simulink model "puzzlebot_controladores"  (R2024a)
settings: Solver=VariableStepAuto  StartTime=0.0  StopTime=220  RelTol=1e-3
libraries: slpidlib x2
settings Model: Creator=KALED  LastModifiedBy=KALED

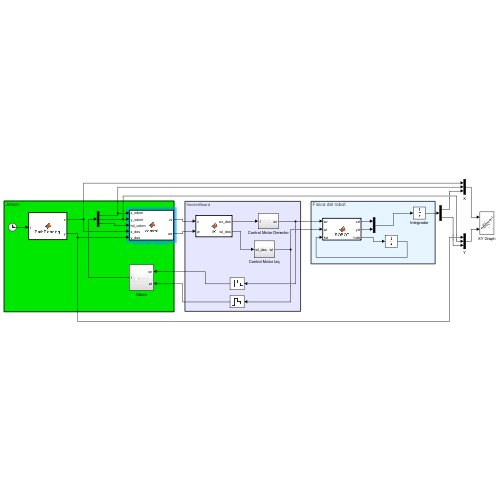
[thumbnail: Simulink's stored preview of the top-level diagram]
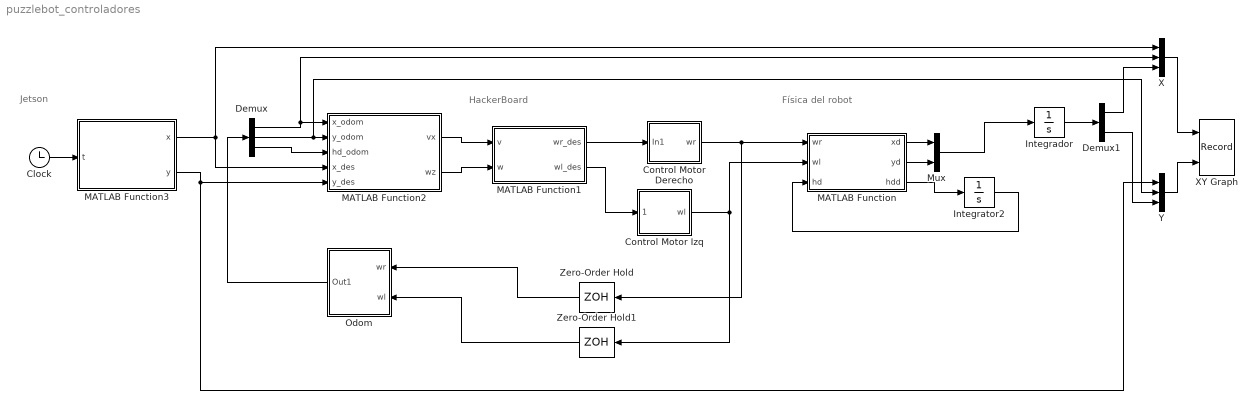
== system puzzlebot_controladores ==
  note: Jetson
  note: HackerBoard
  note: Física del robot
  Clock : Clock
  Control Motor Derecho : Subsystem
  Control Motor Izq : Subsystem
  Demux : Demux  Outputs=3
  Demux1 : Demux  Outputs=2
  Integrador : Integrator  InitialCondition=[0,0]
  Integrator2 : Integrator  ContinuousStateAttributes='orientation'
  MATLAB Function : MATLAB Function  TreatAsAtomicUnit=on
  MATLAB Function1 : MATLAB Function  TreatAsAtomicUnit=on
  MATLAB Function2 : MATLAB Function  TreatAsAtomicUnit=on
  MATLAB Function3 : MATLAB Function  TreatAsAtomicUnit=on
  Mux : Mux  Inputs=2
  Odom : Subsystem
  X : Mux  Inputs=3
  XY Graph : Record  FileSettingsInternal="{\"entries\":[{\"content\":{\"excelSettings\":{\"content\":{},\"type\":\"Streamout.ExcelSettings\"}},\"type\":\"Streamout.FileSettingStorage\",\"uuid\":\"\"}],\"packageUris\":[\"http:\\/\\/schema.mathworks.com\\/mf0\\/streamout_blocks\\/R2020a\"],\"version\":\"1.0\"}"  Layout=[1 1]  SignalsInternal="{\"entries\":[{\"content\":{\"signals\":[{\"content\":{\"blockPath\":[],\"dimensions\":[3],\"domain\":\"\",\"hasChildren\":true,\"lineColor\":\"#fe330a\",\"lineWidth\":2,\"port\":1,\"sid\":[\"\"],\"signalID\":1,\"signalName\":\"X\"},\"type\":\"RecordBlkView.Signal\",\"uuid\":\"\"},{\"content\":{\"blockPath\":[],\"channel\":[1],\"dimensions\":[3],\"domain\":\"\",\"lineColor\":\"#139fff\",\"parentID\":1,\"plots\":[ 1 ],\"port\":1,\"sid\":[\"\"],\"signalID\":2,\"signalName\":\"X\"},\"type\":\"RecordBlkView.Signal\",\"uuid\":\"\"},{\"content\":{\"blockPath\":[],\"dimensions\":[3],\"domain\":\"\",\"hasChildren\":true,\"lineColor\":\"#0072bd\",\"lineWidth\":2,\"port\":2,\"sid\":[\"\"],\"signalID\":3,\"signalName\":\"Y\"},\"type\":\"RecordBlkView.Signal\",\"uuid\":\"\"},{\"content\":{\"blockPath\":[],\"channel\":[1],\"dimensions\":[3],\"domain\":\"\",\"lineColor\":\"#b746ff\",\"parentID\":3,\"plots\":[ 1 ],\"port\":2,\"sid\":[\"\"],\"signalID\":4,\"signalName\":\"Y\"},\"type\":\"RecordBlkView.Signal\",\"uuid\":\"\"},{\"content\":{\"blockPath\":[],\"channel\":[2],\"dimensions\":[3],\"domain\":\"\",\"lineColor\":\"#64d413\",\"parentID\":1,\"plots\":[ 1 ],\"port\":1,\"sid\":[\"\"],\"signalID\":5,\"signalName\":\"X\"},\"type\":\"RecordBlkView.Signal\",\"uuid\":\"\"},{\"content\":{\"blockPath\":[],\"channel\":[3],\"dimensions\":[3],\"domain\":\"\",\"lineColor\":\"#ff6929\",\"lineWidth\":2,\"parentID\":1,\"plots\":[ 1 ],\"port\":1,\"sid\":[\"\"],\"signalID\":6,\"signalName\":\"X\"},\"type\":\"RecordBlkView.Signal\",\"uuid\":\"\"},{\"content\":{\"blockPath\":[],\"channel\":[2],\"dimensions\":[3],\"domain\":\"\",\"lineColor\":\"#ff13a6\",\"parentID\":3,\"plots\":[ 1 ],\"port\":2,\"sid\":[\"\"],\"signalID\":7,\"signalName\":\"Y\"},\"type\":\"RecordBlkView.Signal\",\"uuid\":\"\"},{\"content\":{\"blockPath\":[],\"channel\":[3],\"dimensions\":[3],\"domain\":\"\",\"lineColor\":\"#64d413\",\"lineWidth\":2,\"parentID\":3,\"plots\":[ 1 ],\"port\":2,\"sid\":[\"\"],\"signalID\":8,\"signalName\":\"Y\"},\"type\":\"RecordBlkView.Signal\",\"uuid\":\"\"}]},\"type\":\"RecordBlkView.InputSignals\",\"uuid\":\"\"}],\"packageUris\":[\"http:\\/\\/schema.mathworks.com\\/mf0\\/streamout_blocks\\/R2020a\"],\"version\":\"1.0\"}"  VisualizationBindings="{\"xyplotplugin\":{\"info\":[{\"series\":[{\"bindingParametersList\":[{\"parameter\":\"X-Axis\",\"signalID\":6,\"signalName\":\"X(3)\"},{\"parameter\":\"Y-Axis\",\"signalID\":8,\"signalName\":\"Y(3)\"}],\"seriesID\":0},{\"bindingParametersList\":[{\"parameter\":\"X-Axis\",\"signalID\":2,\"signalName\":\"X(1)\"},{\"parameter\":\"Y-Axis\",\"signalID\":4,\"signalName\":\"Y(1)\"}],\"seriesID\":1},{\"bindingParametersList\":[{\"parameter\":\"X-Axis\",\"signalID\":5,\"signalName\":\"X(2)\"},{\"parameter\":\"Y-Axis\",\"signalID\":7,\"signalName\":\"Y(2)\"}],\"seriesID\":2}],\"subplotID\":1}]}}"  CompatibilityTag=XY
  Y : Mux  Inputs=3
  Zero-Order Hold : ZeroOrderHold  SampleTime=0.01
  Zero-Order Hold1 : ZeroOrderHold  SampleTime=0.01
  wires:
  Odom/1(Out1) -> Demux/1
  X/1 -> XY Graph/1
  Demux1/2 -> Y/3
  Demux/2 -> Y/2, MATLAB Function2/2(y_odom)
  Zero-Order Hold/1 -> Odom/1(wr)
  Demux1/1 -> X/3
  MATLAB Function1/2(wl_des) -> Control Motor Izq/1(wl_des)
  MATLAB Function/3(hdd) -> Integrator2/1
  Integrator2/1 -> MATLAB Function/3(hd)
  Control Motor Derecho/1(wr) -> Zero-Order Hold/1, MATLAB Function/1(wr)
  MATLAB Function1/1(wr_des) -> Control Motor Derecho/1(In1)
  MATLAB Function/1(xd) -> Mux/1
  Integrador/1 -> Demux1/1
  MATLAB Function3/1(x) -> X/1, MATLAB Function2/4(x_des)
  MATLAB Function2/2(wz) -> MATLAB Function1/2(w)
  Mux/1 -> Integrador/1
  MATLAB Function3/2(y) -> Y/1, MATLAB Function2/5(y_des)
  Zero-Order Hold1/1 -> Odom/2(wl)
  MATLAB Function2/1(vx) -> MATLAB Function1/1(v)
  Clock/1 -> MATLAB Function3/1(t)
  Demux/3 -> MATLAB Function2/3(hd_odom)
  MATLAB Function/2(yd) -> Mux/2
  Demux/1 -> X/2, MATLAB Function2/1(x_odom)
  Control Motor Izq/1(wl) -> MATLAB Function/2(wl), Zero-Order Hold1/1
  Y/1 -> XY Graph/2

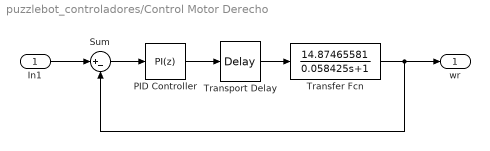
== system puzzlebot_controladores/Control Motor Derecho ==
  In1 : Inport
  PID Controller : slpidlib/PID Controller  Controller=PI  Form=Parallel  TimeDomain=Discrete-time  UseExternalTs=off  SampleTime=0.01  IntegratorMethod=Forward Euler  FilterMethod=Forward Euler  ControllerParametersSource=internal  P=0.03143  I=0.22281  UseKiTs=off  D=0  UseExternalDerivativeSource=off  N=100  UseFilter=on  TunerSelectOption=Transfer Function Based (PID Tuner App)  InitialConditionSource=internal  InitialConditionForIntegrator=0  InitialConditionForFilter=0  DifferentiatorICPrevScaledInput=0  ExternalReset=none  TrackingMode=off  Kt=1  LimitOutput=on  SatLimitsSource=internal  UpperSaturationLimit=1  LowerSaturationLimit=-1  LinearizeAsGain=on  AntiWindupMode=none  Kb=1  LimitIntegrator=off  UpperIntegratorSaturationLimit=inf  LowerIntegratorSaturationLimit=-inf  POutMin=[]  POutMax=[]  IOutMin=[]  IOutMax=[]  DOutMin=[]  DOutMax=[]  NOutMin=[]  NOutMax=[]  SumOutMin=[]  SumOutMax=[]  SaturationOutMin=[]  SaturationOutMax=[]  PParamMin=[]  PParamMax=[]  IParamMin=[]  IParamMax=[]  DParamMin=[]  DParamMax=[]  NParamMin=[]  NParamMax=[]  KbParamMin=[]  KbParamMax=[]  KtParamMin=[]  KtParamMax=[]  KbOutMin=[]  KbOutMax=[]  KtOutMin=[]  KtOutMax=[]  IntegratorOutMin=[]  IntegratorOutMax=[]  FilterOutMin=[]  FilterOutMax=[]  SumI1OutMin=[]  SumI1OutMax=[]  SumI2OutMin=[]  SumI2OutMax=[]  SumI3OutMin=[]  SumI3OutMax=[]  SumI4OutMin=[]  SumI4OutMax=[]  SumDOutMin=[]  SumDOutMax=[]  DifferentiatorOutMin=[]  DifferentiatorOutMax=[]  FilterDiffOutCoefMin=[]  FilterDiffOutCoefMax=[]  ReciprocalOutMin=[]  ReciprocalOutMax=[]  SumDenOutMin=[]  SumDenOutMax=[]  SumNumOutMin=[]  SumNumOutMax=[]  DivideOutMin=[]  DivideOutMax=[]  UdiffTsProdOutMin=[]  UdiffTsProdOutMax=[]  NTsProdOutMin=[]  NTsProdOutMax=[]  UintegralTsProdOutMin=[]  UintegralTsProdOutMax=[]  UngainTsProdOutMin=[]  UngainTsProdOutMax=[]  ClampingZeroOutDataTypeStr=Inherit: Inherit via back propagation  ClampingZeroOutMin=[]  ClampingZeroOutMax=[]  FilterDenConstantOutDataTypeStr=Inherit: Inherit via back propagation  FilterDenConstantOutMin=[]  FilterDenConstantOutMax=[]  PCopyOutDataTypeStr=Inherit: Inherit via back propagation  PCopyOutMin=[]  PCopyOutMax=[]  NCopyOutDataTypeStr=Inherit: Inherit via back propagation  NCopyOutMin=[]  NCopyOutMax=[]  IntegratorContinuousStateAttributes=''  IntegratorStateMustResolveToSignalObject=off  IntegratorRTWStateStorageClass=Auto  FilterContinuousStateAttributes=''  FilterStateMustResolveToSignalObject=off  FilterRTWStateStorageClass=Auto  ParallelPVariant=InternalParameters  IdealPVariant=Disabled  IVariant=InternalParameters  DVariant=Disabled  IntegratorVariant=Discrete  SatVariant=Enabled  AWVariant=Passthrough  PCopyVariant=Disabled  TRVariant=Disabled  FdbkBlocksVariant=Forward  IdealPFdbkVariant=Disabled  SatFdbkVariant=Disabled  DerivativeFilterVariant=Disabled  NVariant=Disabled  NCopyVariant=Disabled_SignalSpec  FilterICVariant=Disabled  IntegratorICVariant=InternalICs  ExternalResetVariant=Disabled  TRSumVariant=Passthrough  SumFdbkVariant=Disabled  SumVariant=Sum_PI  TsampFilterVariant=InternalTs  TsampNgainVariant=Passthrough  TsampIntegralVariant=Disabled_SignalSpec  ExternalSaturationOutDataTypeStr=Inherit: Same as second input  DerivativeSourceVariant=Disabled
  Sum : Sum  Inputs=|+-
  Transfer Fcn : TransferFcn  Numerator=14.87465581  Denominator=[0.058425 1]
  Transport Delay : TransportDelay  DelayTime=0.043735
  wr : Outport
  wires:
  In1/1 -> Sum/1
  Transfer Fcn/1 -> wr/1, Sum/2
  Transport Delay/1 -> Transfer Fcn/1
  Sum/1 -> PID Controller/1
  PID Controller/1 -> Transport Delay/1

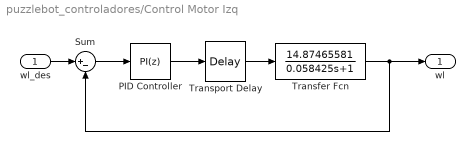
== system puzzlebot_controladores/Control Motor Izq ==
  wl_des : Inport
  PID Controller : slpidlib/PID Controller  Controller=PI  Form=Parallel  TimeDomain=Discrete-time  UseExternalTs=off  SampleTime=0.01  IntegratorMethod=Forward Euler  FilterMethod=Forward Euler  ControllerParametersSource=internal  P=0.03143  I=0.22281  UseKiTs=off  D=0  UseExternalDerivativeSource=off  N=100  UseFilter=on  TunerSelectOption=Transfer Function Based (PID Tuner App)  InitialConditionSource=internal  InitialConditionForIntegrator=0  InitialConditionForFilter=0  DifferentiatorICPrevScaledInput=0  ExternalReset=none  TrackingMode=off  Kt=1  LimitOutput=off  SatLimitsSource=internal  UpperSaturationLimit=inf  LowerSaturationLimit=-inf  LinearizeAsGain=on  AntiWindupMode=none  Kb=1  LimitIntegrator=off  UpperIntegratorSaturationLimit=inf  LowerIntegratorSaturationLimit=-inf  POutMin=[]  POutMax=[]  IOutMin=[]  IOutMax=[]  DOutMin=[]  DOutMax=[]  NOutMin=[]  NOutMax=[]  SumOutMin=[]  SumOutMax=[]  SaturationOutMin=[]  SaturationOutMax=[]  PParamMin=[]  PParamMax=[]  IParamMin=[]  IParamMax=[]  DParamMin=[]  DParamMax=[]  NParamMin=[]  NParamMax=[]  KbParamMin=[]  KbParamMax=[]  KtParamMin=[]  KtParamMax=[]  KbOutMin=[]  KbOutMax=[]  KtOutMin=[]  KtOutMax=[]  IntegratorOutMin=[]  IntegratorOutMax=[]  FilterOutMin=[]  FilterOutMax=[]  SumI1OutMin=[]  SumI1OutMax=[]  SumI2OutMin=[]  SumI2OutMax=[]  SumI3OutMin=[]  SumI3OutMax=[]  SumI4OutMin=[]  SumI4OutMax=[]  SumDOutMin=[]  SumDOutMax=[]  DifferentiatorOutMin=[]  DifferentiatorOutMax=[]  FilterDiffOutCoefMin=[]  FilterDiffOutCoefMax=[]  ReciprocalOutMin=[]  ReciprocalOutMax=[]  SumDenOutMin=[]  SumDenOutMax=[]  SumNumOutMin=[]  SumNumOutMax=[]  DivideOutMin=[]  DivideOutMax=[]  UdiffTsProdOutMin=[]  UdiffTsProdOutMax=[]  NTsProdOutMin=[]  NTsProdOutMax=[]  UintegralTsProdOutMin=[]  UintegralTsProdOutMax=[]  UngainTsProdOutMin=[]  UngainTsProdOutMax=[]  ClampingZeroOutDataTypeStr=Inherit: Inherit via back propagation  ClampingZeroOutMin=[]  ClampingZeroOutMax=[]  FilterDenConstantOutDataTypeStr=Inherit: Inherit via back propagation  FilterDenConstantOutMin=[]  FilterDenConstantOutMax=[]  PCopyOutDataTypeStr=Inherit: Inherit via back propagation  PCopyOutMin=[]  PCopyOutMax=[]  NCopyOutDataTypeStr=Inherit: Inherit via back propagation  NCopyOutMin=[]  NCopyOutMax=[]  IntegratorContinuousStateAttributes=''  IntegratorStateMustResolveToSignalObject=off  IntegratorRTWStateStorageClass=Auto  FilterContinuousStateAttributes=''  FilterStateMustResolveToSignalObject=off  FilterRTWStateStorageClass=Auto  ParallelPVariant=InternalParameters  IdealPVariant=Disabled  IVariant=InternalParameters  DVariant=Disabled  IntegratorVariant=Discrete  SatVariant=Disabled  AWVariant=Passthrough  PCopyVariant=Disabled  TRVariant=Disabled  FdbkBlocksVariant=Forward  IdealPFdbkVariant=Disabled  SatFdbkVariant=Disabled  DerivativeFilterVariant=Disabled  NVariant=Disabled  NCopyVariant=Disabled_SignalSpec  FilterICVariant=Disabled  IntegratorICVariant=InternalICs  ExternalResetVariant=Disabled  TRSumVariant=Passthrough  SumFdbkVariant=Disabled  SumVariant=Sum_PI  TsampFilterVariant=InternalTs  TsampNgainVariant=Passthrough  TsampIntegralVariant=Disabled_SignalSpec  ExternalSaturationOutDataTypeStr=Inherit: Same as second input  DerivativeSourceVariant=Disabled
  Sum : Sum  Inputs=|+-
  Transfer Fcn : TransferFcn  Numerator=14.87465581  Denominator=[0.058425 1]
  Transport Delay : TransportDelay  DelayTime=0.043735
  wl : Outport
  wires:
  Sum/1 -> PID Controller/1
  PID Controller/1 -> Transport Delay/1
  Transfer Fcn/1 -> wl/1, Sum/2
  Transport Delay/1 -> Transfer Fcn/1
  wl_des/1 -> Sum/1

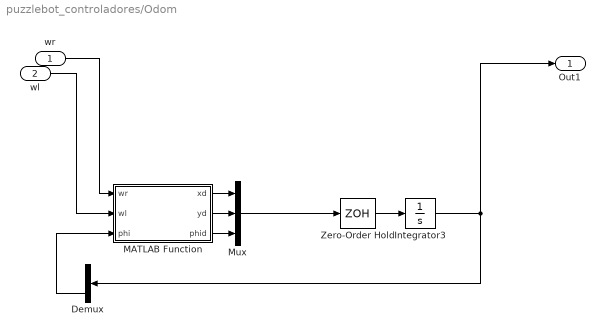
== system puzzlebot_controladores/Odom ==
  wr : Inport
  wl : Inport  Port=2
  Demux : Demux  Outputs=3
  Integrator3 : Integrator  InitialCondition=[0,0,0]
  MATLAB Function : MATLAB Function  TreatAsAtomicUnit=on
  Mux : Mux  Inputs=3
  Zero-Order Hold : ZeroOrderHold  SampleTime=0.01
  Out1 : Outport
  wires:
  Mux/1 -> Zero-Order Hold/1
  wl/1 -> MATLAB Function/2(wl)
  Integrator3/1 -> Demux/1, Out1/1
  Zero-Order Hold/1 -> Integrator3/1
  wr/1 -> MATLAB Function/1(wr)
  MATLAB Function/1(xd) -> Mux/1
  MATLAB Function/2(yd) -> Mux/2
  MATLAB Function/3(phid) -> Mux/3
  Demux/3 -> MATLAB Function/3(phi)

== matlab function puzzlebot_controladores/MATLAB Function1 ==
  data: v input; wr_des output; w input; wl_des output
function [wr_des,wl_des] = IK(v,w) % Twist local
% des se refiere a deseada. 
% Vx es la velocidad en x y wz es la velocidad angular en Z
R=0.0505;
b=0.1712;

wr_des=(v/R)+(w*b/(2*R));
wl_des=(v/R)-(w*b/(2*R));

== matlab function puzzlebot_controladores/MATLAB Function ==
  data: wr input; xd output; wl input; hd input; yd output; hdd output
function [xd, yd, hdd] = ROBOT(wr,wl,hd) %hd es heading
% Heading es la dirección de movimiento y es letra griega phi
% Las letras latinas son translacionales y letras griegas son rotacionales
% El sufijo d en xd yd y hdd es por derivada (Se transforma en velocidad)
% Además xd yd hdd están en el sistema de referencia fijo

R=0.0505;%Metros
b=0.1712; %Metros

xd= (wr+wl)*(R/2)*cos(hd); %Vxl*Cos(phi)
yd= (wr+wl)*(R/2)*sin(hd); %Vxl*Sin(phi)
hdd=(wr-wl)*(R/b);

== matlab function puzzlebot_controladores/MATLAB Function2 ==
  data: x_odom input; vx output; y_odom input; hd_odom input; wz output; x_des input; y_des input
function [vx, wz] = control(x_odom, y_odom, hd_odom, x_des, y_des)

% Parámetros del controlador
Kl = 1;     % Ganancia proporcional para posición (modo 1 y 2)
Kw = 1.52;  % Ganancia proporcional para orientación

% Definir el modo de control:
% 1 = Turn while go
% 2 = Turn then go
% 3 = Lyapunov
% 4 = Pure Pursuit
modo = 3;

% Errores calculados
dx = x_des - x_odom;
dy = y_des - y_odom;
e_pos = sqrt(dx^2 + dy^2);
hd_des = atan2(dy, dx);
e_ori = hd_des - hd_odom;
e_ori_norm = atan2(sin(e_ori), cos(e_ori));  % Normalizar error de orientación

switch modo
    case 1  % Turn while go
        if e_pos < 0.01
            vx = 0;
            wz = 0;
        else
            if abs(e_ori_norm) > pi/4 % 45 Grados
                vx = min(e_pos * Kl * 0.3, 0.2); % reduce velocidad
            else
                vx = min(e_pos * Kl, 0.2);
            end

            if abs(e_ori_norm) < deg2rad(1)
                wz = 0;
            else
                wz = max(min(e_ori_norm * Kw, 0.2), -0.2);
            end
        end

    case 2  % Turn then go
        if abs(e_ori_norm) > deg2rad(1)
            vx = 0;
            wz = max(min(e_ori_norm * Kw, 0.2), -0.2);
        elseif e_pos > 0.01
            wz = 0;
            vx = min(e_pos * Kl, 0.2);
        else
            vx = 0;
            wz = 0;
        end

    case 3  % Lyapunov Control
        k1 = 2.0;  % Aumenta para lograr wz cercanos a 0.6
        k2 = 1.0;
    
        % Velocidad de referencia (limitada a 0.2 m/s)
        v_r = min(0.2, 0.5 * e_pos);
        vx = v_r * cos(e_ori_norm);
    
        % Corrección angular Lyapunov
        if abs(e_ori_norm) > 1e-3
            correction = (v_r * cos(e_ori_norm) * sin(e_ori_norm) * (e_ori_norm + k2 * hd_des)) / e_ori_norm;
        else
            correction = 0;
        end
    
        wz = k1 * e_ori_norm + correction;
    
        % Saturación angular
        wz = max(min(wz, 0.6), -0.6);
    
        if e_pos < 0.05
            vx = 0;
            wz = 0;
        end


    case 4  % Pure Pursuit
        L = 0.6;  % Lookahead distance (ajustable)
        v = min(0.2, e_pos);  % Velocidad proporcional a la distancia

        % Error lateral (suponiendo robot como punto) proyectado en eje lateral local
        y_r = -sin(hd_odom) * dx + cos(hd_odom) * dy;

        % Cálculo de la curvatura
        kappa = (2 * y_r) / (L^2);
        wz = v * kappa;
        vx = v;

        % Detención si está cerca del objetivo
        if e_pos < 0.05
            vx = 0;
            wz = 0;
        end
end

== matlab function puzzlebot_controladores/Odom/MATLAB Function ==
  data: wr input; xd output; wl input; phi input; yd output; phid output
function [xd, yd, phid] = cinematica(wr,wl,phi) %Psi es el heading.
% El heading es la orientación (dirección del mov)
% Las letras latina son translacionales, las letras griegas son
% rotacionales)
%El sufijo d significa (derivada) (Lo transforma en velocidad)

R=0.0505;%Metros
b=0.1712; %Metros

xd= (wr+wl)*(R/2)*cos(phi); %Vxl*Cos(phi)
yd= (wr+wl)*(R/2)*sin(phi); %Vxl*Sin(phi)
phid=(wr-wl)*(R/b);

== matlab function puzzlebot_controladores/MATLAB Function3 ==
  data: x output; t input; y output
function [x, y] = PathPlanning(t)

% Se cambia seno y coseno debido a la orientación y el desplazamiento 
% de las funciones como coseno desplazado pi/2 es seno
%x = r*sin(w*t)
    if t < 60
        x = 2; y = 2;     % Cuadrante I
    elseif t < 120
        x = -2; y = 2;    % Cuadrante II
    elseif t < 180
        x = -2; y = -2;   % Cuadrante III
    elseif t < 240
        x = 2; y = -2;    % Cuadrante IV
    else
        x = 0; y = 0;     % Regresa al origen
    end
end
